simulink model "single_engine_kalman"  (R2018b)
settings: Solver=VariableStepAuto  StartTime=0.0  StopTime=10.0  FixedStep=0.001  RelTol=1e-3
values from neighbouring files (symbols this model uses):
  A = J*(Omega_phi + Omega)    [IMU.m]
  D = simplify(D)    [dynamika_gimbala_symbolicznie.m]    (also in dynamika_gimbala_symbolicznie_20190706.m; dynamika_gimbala_symbolicznie_20190825.m; gimbal_dynamics.m = calculate_D_matrix(THETA,I1,I2,I3,DIM))
  R = 7.9    [BLDC_simulator.m]    (also in engine_parameters.m; engine_parameters_20191210.m = 0.5; inversekinematics.m = Rg*Rd*Rm)
undefined symbols (not defined in the file or in its folder): B, C, Continuous, Time
libraries: ctrlSharedLib x1
settings Model: Creator=Paweł Tymiński  LastModifiedBy=Paweł Tymiński

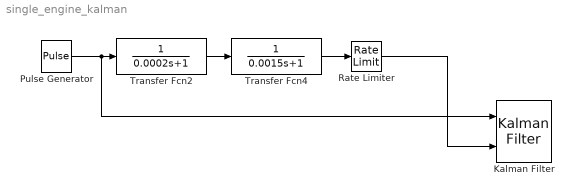
== system single_engine_kalman ==
  Kalman Filter : ctrlSharedLib/Kalman Filter  TimeDomain=Continuous-Time  UseCurrentEstimator=on  ModelSource=Individual A, B, C, D matrices  ModelSourceVariable=ss(0.95,1,1,0,1)  A=A  B=B  C=C  D=D  NumberOfStates=1  NumberOfInputs=1  NumberOfOutputs=1  InitialEstimateSource=Dialog  X0=0  P0=10  UseK=off  UseGH=off  NumberOfProcessNoiseInputs=1  G=1  TimeInvariantG=on  H=0  TimeInvariantH=on  Q=Q  TimeInvariantQ=on  R=R  TimeInvariantR=on  N=0  TimeInvariantN=on  AddInputPort=on  AddEnablePort=off  OutputEstimatedY=on  OutputP=off  Ts=-1
      settings: SourceProductBaseCode=CT
  Pulse Generator : DiscretePulseGenerator  PulseType=Time based  Period=1  PulseWidth=10
  Rate Limiter : RateLimiter  RisingSlewLimit=18.5  FallingSlewLimit=-18.5  SampleTimeMode=inherited
  Transfer Fcn2 : TransferFcn  Denominator=[0.0002 1]
  Transfer Fcn4 : TransferFcn  Denominator=[0.0015 1]
  wires:
  Rate Limiter/1 -> Kalman Filter/2
  Transfer Fcn4/1 -> Rate Limiter/1
  Pulse Generator/1 -> Kalman Filter/1, Transfer Fcn2/1
  Transfer Fcn2/1 -> Transfer Fcn4/1
